simulink model "simlink_TCG"  (R2021a)
settings: Solver=VariableStepAuto  StartTime=0.0  StopTime=500  RelTol=1e-6
settings Model: Creator=l_w_h  LastModifiedBy=l_w_h
settings SolverCC: AlgebraicLoopSolver=TrustRegion

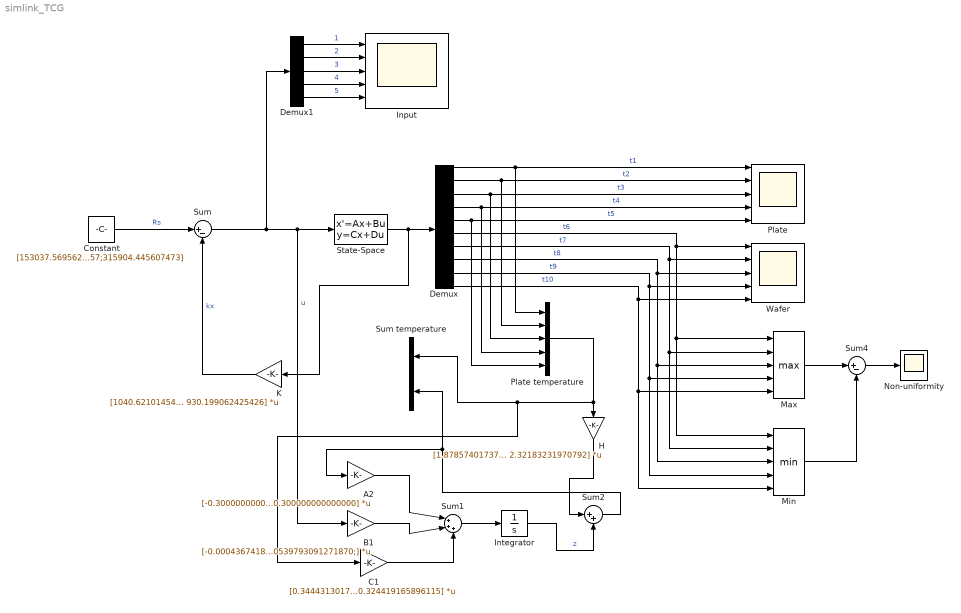
== system simlink_TCG ==
  A2 : Gain  Gain=[-0.300000000000000 0 0 0 0;0 -0.300000000000000 -6.93889390390723e-18 0 0;0 6.93889390390723e-18 -0.300000000000000 0 0;0 0 0 -0.300000000000000 6.93889390390723e-18;0 0 0 -3.46944695195361e-18 -0.300000000000000]  Multiplication=Matrix(K*u)
  B1 : Gain  Gain=[-0.000436741821281746 -0.000201465857250265 0 0 0;-6.71552857500885e-05 -0.000426624199007793 -0.000144428193774131 0 0;0 -8.66569162644783e-05 -0.000419989912703969 -0.000131560849563564 0;0 0 -9.39720354025459e-05 -0.000418421215569420 -0.000125814427560046;0 0 0 -9.78556658800356e-05 -0.000539793091271870;]  Multiplication=Matrix(K*u)
  C1 : Gain  Gain=[0.344431301747057 -0.0117512821095320 -0.0385532259236173 0 0;-0.00391709403651067 0.328438474570554 -0.00521863281406086 -0.0251759540060748 0;-0.00771064518472346 -0.00313117968843653 0.330223715802212 -0.00332379586198954 -0.0219313013531552;0 -0.0107896945740321 -0.00237413990142110 0.330533705208892 -0.0231878429325686;0 0 -0.0121840563073084 -0.0180054811749444 0.324419165896115]  Multiplication=Matrix(K*u)
  Constant : Constant  Value=[153037.569562540;-33139.2843468048;45321.8245165428;210076.349949157;315904.445607473]
  Demux : Demux  Outputs=10
  Demux1 : Demux  Outputs=5
  H : Gain  Gain=[1.87857401737166 0.866572666906799 0 0 0;0.288857555635600 1.83505470826210 0.621234420380753 0 0;0 0.372740652228452 1.80651840313430 0.565887628915702 0;0 0 0.404205449225502 1.79977090716645 0.541170327886501;0 0 0 0.420910255022834 2.32183231970792]  Multiplication=Matrix(K*u)
  Input : Scope  NumInputPorts=5
  Integrator : Integrator
  K : Gain  Gain=[1040.62101454270 -320.306170322634 -59.2252313244026 227.958918565248 240.894856638426 372.138527897946 -370.696546217003 -193.562742645483 152.368074523857 243.750083253837;-395.036959442210 1445.41180545318 3.18106966337142 -126.523424745173 -46.0693531161156 -197.976432827956 288.642703261052 -443.711626792953 -527.966761706448 -347.879849156491;294.427032872561 98.6952411671996 1588.82433574057 -141.789308987864 -339.372732658242 341.777038896890 -153.758096629279 107.707837102094 -667.340837544668 -789.363065136329;587.380771783650 155.141189560613 -169.824494221811 1583.13935792459 -76.7995719465899 561.593808476052 -42.8157476374401 -615.451553335194 230.179830245042 -399.152672685820;560.472995294831 202.481930994585 -293.202114526122 -151.636707732806 2026.73913099616 521.004981087144 58.6334649325038 -640.258411444693 -453.015908658764 930.199062425426]  Multiplication=Matrix(K*u)
  Max : MinMax  Function=max  Inputs=5
  Min : MinMax  Inputs=5
  Non-uniformity : Scope
  Plate : Scope  NumInputPorts=5
  Plate temperature : Mux  Inputs=5
  State-Space : StateSpace  A=[-0.117855659679215 0.0620590628252506 0 0 0 0.0557965968539647 0 0 0 0;0.0206863542750835 -0.120972267946796 0.0444893168177479 0 0 0 0.0557965968539647 0 0 0;0 0.0266935900906488 -0.123015877698588 0.0405256907539742 0 0 0 0.0557965968539647 0 0;0 0 0.0289469219671245 -0.123499095427663 0.0387555766065743 0 0 0 0.0557965968539647 0;0 0 0 0.0301432262495578 -0.0860418872487965 0 0 0 0 0.0557965968539647;0.140956950866225 0 0 0 0 -0.195181962892381 0.0483518057400637 0 0 0;0 0.140956950866225 0 0 0 0.0161172685800212 -0.197610192238130 0.0346627665057913 0 0;0 0 0.140956950866225 0 0 0 0.0207976599034748 -0.199202420951047 0.0315746038952554 0;0 0 0 0.140956950866225 0 0 0 0.0225532884966110 -0.199578908263339 0.0301954626144110;0 0 0 0 0.140956950866225 0 0 0 0.0234853598112085 -0.170449658094751]  B=[0.000232485820224853 0 0 0 0;0 0.000232485820224853 0 0 0;0 0 0.000232485820224853 0 0;0 0 0 0.000232485820224853 0;0 0 0 0 0.000232485820224853;0 0 0 0 0;0 0 0 0 0;0 0 0 0 0;0 0 0 0 0;0 0 0 0 0]  C=[1 0 0 0 0 0 0 0 0 0;0 1 0 0 0 0 0 0 0 0;0 0 1 0 0 0 0 0 0 0;0 0 0 1 0 0 0 0 0 0;0 0 0 0 1 0 0 0 0 0;0 0 0 0 0 1 0 0 0 0;0 0 0 0 0 0 1 0 0 0;0 0 0 0 0 0 0 1 0 0;0 0 0 0 0 0 0 0 1 0;0 0 0 0 0 0 0 0 0 1]  D=[0 0 0 0 0;0 0 0 0 0;0 0 0 0 0;0 0 0 0 0;0 0 0 0 0;0 0 0 0 0;0 0 0 0 0;0 0 0 0 0;0 0 0 0 0;0 0 0 0 0]  InitialCondition=[114.583333333333;114.583333333333;114.583333333333;114.583333333333;114.688014403292;25;25;25;25;25]
  Sum : Sum  Inputs=|+-
  Sum temperature : Mux  Inputs=2
  Sum1 : Sum  Inputs=|+++
  Sum2 : Sum  Inputs=|++
  Sum4 : Sum  Inputs=|+-
  Wafer : Scope  NumInputPorts=5
  wires:
  Demux/5 -> Plate/5, Plate temperature/5  "t5"
  Demux/3 -> Plate/3, Plate temperature/3  "t3"
  Demux/1 -> Plate/1, Plate temperature/1  "t1"
  Demux/2 -> Plate/2, Plate temperature/2  "t2"
  Demux/4 -> Plate/4, Plate temperature/4  "t4"
  Sum/1 -> Demux1/1, B1/1, State-Space/1  "u"
  Plate temperature/1 -> C1/1, Sum temperature/1, H/1
  A2/1 -> Sum1/1
  C1/1 -> Sum1/3
  Sum1/1 -> Integrator/1
  K/1 -> Sum/2  "kx"
  Max/1 -> Sum4/1
  Min/1 -> Sum4/2
  Sum4/1 -> Non-uniformity/1
  Demux1/1 -> Input/1  "1"
  Demux1/2 -> Input/2  "2"
  Demux1/3 -> Input/3  "3"
  Demux1/4 -> Input/4  "4"
  Demux1/5 -> Input/5  "5"
  State-Space/1 -> K/1, Demux/1
  Constant/1 -> Sum/1  "Rs"
  Demux/6 -> Wafer/1, Max/1, Min/1  "t6"
  Demux/7 -> Wafer/2, Max/2, Min/2  "t7"
  Demux/8 -> Wafer/3, Max/3, Min/3  "t8"
  Demux/9 -> Wafer/4, Max/4, Min/4  "t9"
  Demux/10 -> Wafer/5, Max/5, Min/5  "t10"
  Integrator/1 -> Sum2/2  "z"
  H/1 -> Sum2/1
  Sum2/1 -> A2/1, Sum temperature/2
  B1/1 -> Sum1/2
